simulink model "WT_SP_model_vs1total"  (R2019a)
settings: Solver=ode45  StartTime=0.0  StopTime=365*3600*24  MaxStep=900  RelTol=1e-3
InitFcn:
  | global Az Inc
  | Setup_Toutdoor
  | Setup_qsolar2
  | Setup_wind
  | load SOL
  | load Toutdoor
  | load wind
settings Model: Creator=actaal  LastModifiedBy=actaal
settings DataIOCC: SaveFormat=Array  ReturnWorkspaceOutputs=off
settings OptimizationCC: BlockReduction=off  BooleanDataType=off  LifeSpan=inf
settings DebuggingCC: SaveWithParameterizedLinksMsg=none  UnderspecifiedInitializationDetection=Classic  MergeDetectMultiDrivingBlocksExec=none  SignalResolutionControl=TryResolveAllWithWarning  SFUnexpectedBacktrackingDiag=warning  SFNoUnconditionalDefaultTransitionDiag=warning  SFExecutionAtInitializationDiag=none  ArithmeticOperatorsInVariantConditions=warning
settings HardwareCC: ProdBitPerPointer=32  ProdBitPerSizeT=32  ProdBitPerPtrDiffT=32  ProdLargestAtomicFloat=None  ProdIntDivRoundTo=Undefined  ProdEndianess=Unspecified  ProdWordSize=32  ProdHWDeviceType=32-bit Generic  TargetUnknown=on
settings ModelReferenceCC: PropagateSignalLabelsOutOfModel=off
settings SFSimCC: SimUseLocalCustomCode=off
settings RTWCC: RTWUseLocalCustomCode=off
settings CodeAppCC: StateflowObjectComments=on
settings GRTTargetCC: TargetLangStandard=C89/C90 (ANSI)  GeneratePreprocessorConditionals=Disable all
settings ConfigComp: CovMetricSettings=dw  CovHtmlReporting=on  CovSaveCumulativeToWorkspaceVar=on  CovSaveSingleToWorkspaceVar=on  CovExternalEMLEnable=off  CovSFcnEnable=off

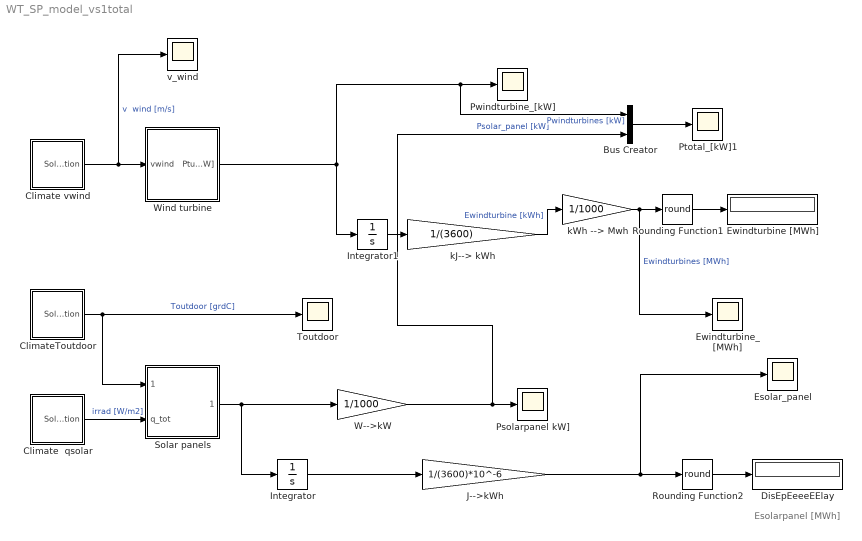
== system WT_SP_model_vs1total ==
  note: Esolarpanel [MWh]
  Bus Creator : BusCreator  Inputs=2
  Climate  qsolar : Subsystem
      mask init:
      | %global Az Inc
      | %Setup_qsolar
      | %load SOL
      mask Display: disp('qsolar')
  Climate vwind : Subsystem
      mask init:
      | %global Az Inc
      | %Setup_qsolar
      | %load SOL
      mask Display: disp('vwind')
  ClimateToutdoor : Subsystem
      mask init:
      | %global Az Inc
      | %Setup_qsolar
      | %load SOL
      mask Display: disp('Toutdoor')
  DisEpEeeeEElay : Display
      settings: Description=Esolar
  Esolar_panel : Scope
  Ewindturbine [MWh] : Display
      settings: Description=Esolar
  Ewindturbine_[MWh] : Scope
  Integrator : Integrator
  Integrator1 : Integrator
  J-->kWh : Gain  Gain=1/(3600)*10^-6
  Psolarpanel kW] : Scope
  Ptotal_[kW]1 : Scope
  Pwindturbine_[kW] : Scope
  Rounding Function1 : Rounding  Operator=round
  Rounding Function2 : Rounding  Operator=round
  Solar panels : Subsystem  mask(Component){ethasp=15, Opp=10000,0,0,0, Az=0,0,0,0, Inc=15,15,45,0}
      mask prompts: ethasp "Efficiency [%]"; Opp "Surface [m2]"; Az "Azimuth [0..360, 0 = south]"; Inc "Inclination [0..90, 0 = horizontal]"
      mask help:
      | Total electricity by solar panels
      | Input in de form of a vector: x, y, z
      mask init:
      | clear global Az Inc
      | Az = str2num(Az);
      | Inc = str2num(Inc);
      | Opp = str2num(Opp);
      | global Az Inc
      mask Help:
      | This model calculates the supplied electricity by a set of solar panels.
      | It is a simple model because the efficiency of all panels has a constant value
      | and the influence of the outdoor temperature is neglected.
      mask Display: disp('Solar panel')
  Toutdoor : Scope
  W-->kW : Gain  Gain=1/1000
  Wind turbine : Subsystem  mask(Component){P=[0 0 10 80 160 300 400 400 400], v=[0 1 2 4 6 8 10 20 30], h=10, a=1, nwt=2}
      mask prompts: P "Power [kW]"; v "Wind velocity [m/s]"; h "Hoogte rotoras [m]"; a "Terreingesteldheid a"; nwt "Aantal turbines"
      mask help:
      | Total electricity by solar panels
      | Input in de form of a vector: x, y, z
      mask Help:
      | This model calculates the supplied electricity by a set of solar panels.
      | It is a simple model because the efficiency of all panels has a constant value
      | and the influence of the outdoor temperature is neglected.
      mask Display:
      | %image('vertrekpic.jpg')
      | disp('Wind turbine')
  kJ--> kWh : Gain  Gain=1/(3600)
  kWh --> Mwh : Gain  Gain=1/1000
  v_wind : Scope
  wires:
  Climate  qsolar/1(Solar radiation) -> Solar panels/2(q_tot)  "irrad [W/m2]"
  Solar panels/1(qsolar [W]) -> Integrator/1, W-->kW/1
  Integrator/1 -> J-->kWh/1
  ClimateToutdoor/1(Solar radiation) -> Solar panels/1(Toutdoor), Toutdoor/1  "Toutdoor [grdC]"
  Climate vwind/1(Solar radiation) -> v_wind/1, Wind turbine/1(vwind)  "v  wind [m/s]"
  Integrator1/1 -> kJ--> kWh/1
  Rounding Function1/1 -> Ewindturbine [MWh]/1
  kWh --> Mwh/1 -> Ewindturbine_[MWh]/1, Rounding Function1/1  "Ewindturbines [MWh]"
  W-->kW/1 -> Bus Creator/2, Psolarpanel kW]/1  "Psolar_panel [kW]"
  Wind turbine/1(Pturb [kW]) -> Bus Creator/1, Pwindturbine_[kW]/1, Integrator1/1  "Pwindturbines [kW]"
  Rounding Function2/1 -> DisEpEeeeEElay/1
  J-->kWh/1 -> Rounding Function2/1, Esolar_panel/1
  kJ--> kWh/1 -> kWh --> Mwh/1  "Ewindturbine [kWh]"
  Bus Creator/1 -> Ptotal_[kW]1/1

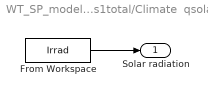
== system WT_SP_model_vs1total/Climate  qsolar ==
  From Workspace : FromWorkspace  VariableName=Irrad  SampleTime=0
  Solar radiation : Outport
  wires:
  From Workspace/1 -> Solar radiation/1

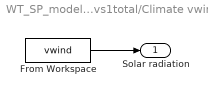
== system WT_SP_model_vs1total/Climate vwind ==
  From Workspace : FromWorkspace  VariableName=vwind  SampleTime=0
  Solar radiation : Outport
  wires:
  From Workspace/1 -> Solar radiation/1

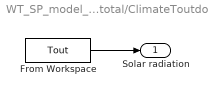
== system WT_SP_model_vs1total/ClimateToutdoor ==
  From Workspace : FromWorkspace  VariableName=Tout  SampleTime=0
  Solar radiation : Outport
  wires:
  From Workspace/1 -> Solar radiation/1

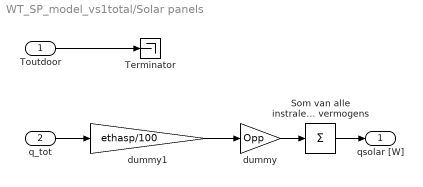
== system WT_SP_model_vs1total/Solar panels ==
  Toutdoor : Inport
  q_tot : Inport  Port=2
  Som van alle instralende vermogens : Sum  Inputs=+
  Terminator : Terminator
  dummy : Gain  Gain=Opp
  dummy1 : Gain  Gain=ethasp/100
  qsolar [W] : Outport
  wires:
  q_tot/1 -> dummy1/1
  dummy/1 -> Som van alle instralende vermogens/1
  Som van alle instralende vermogens/1 -> qsolar [W]/1
  dummy1/1 -> dummy/1
  Toutdoor/1 -> Terminator/1

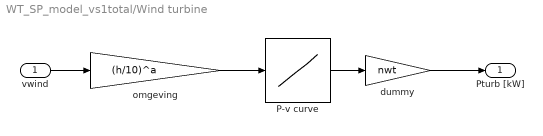
== system WT_SP_model_vs1total/Wind turbine ==
  vwind : Inport
  P-v curve : Lookup_n-D  NumberOfTableDimensions=1  BreakpointsForDimension1=v  Table=P  InternalRulePriority=Speed  RndMeth=Simplest  InputSameDT=on
  dummy : Gain  Gain=nwt
  omgeving : Gain  Gain=(h/10)^a
  Pturb [kW] : Outport
  wires:
  vwind/1 -> omgeving/1
  dummy/1 -> Pturb [kW]/1
  P-v curve/1 -> dummy/1
  omgeving/1 -> P-v curve/1
